simulink model "torch_3dof_angle"  (R2024a)
settings: Solver=FixedStepAuto  StartTime=0.0  StopTime=50  FixedStep=framePeriod_s  RelTol=1e-3
undefined symbols (not defined in the file): Aircraft, DiscIntNeverNeededParam, framePeriod_s, frameRate_hz, magnitude
libraries: simulink x36, slpidlib x11, dspmathops x1, simulink_extras x1
(part 3 of 4)

== system torch_3dof_angle/WAYPOINT CONTROLLER/WP_NAV/Subsystem ==
  Sys_input : Inport
  tar_pos : Inport  Port=2
  max_v_z_mps : Inport  Port=3
  Bus Selector : BusSelector  OutputSignals=StateEstData.aux_ins.ned_pos_m
  Cast To Single : DataTypeConversion  OutDataTypeStr=single  SaturateOnIntegerOverflow=off  RndMeth=Floor
  Selector : Selector  InputPortWidth=3  IndexOptions=Index vector (dialog)  Indices=3  OutputSizes=1
  Selector1 : Selector  InputPortWidth=3  IndexOptions=Index vector (dialog)  Indices=3  OutputSizes=1
  Vertical position controller1 : Subsystem
  ve_z_cmd_mps : Outport
  wires:
  Vertical position controller1/1(ve_z_cmd_mps) -> ve_z_cmd_mps/1  "ve_z_cmd_mps"
  tar_pos/1 -> Selector/1
  Sys_input/1 -> Bus Selector/1
  Bus Selector/1 -> Selector1/1  "<ned_pos_m>"
  Selector1/1 -> Cast To Single/1
  max_v_z_mps/1 -> Vertical position controller1/3(max_v_z_mps)
  Selector/1 -> Vertical position controller1/2(tar_z)
  Cast To Single/1 -> Vertical position controller1/1(cur_alt)

== system torch_3dof_angle/WAYPOINT CONTROLLER/WP_NAV/Vertical position controller ==
  Sys_input : Inport
  max_v_z_mps : Inport  Port=2
  cur_target_pos_m : Inport  Port=3
  Bus Selector6 : BusSelector  OutputSignals=Navigation Filter Data.bfs_ekf.ned_pos_m
  Selector1 : Selector  InputPortWidth=3  IndexOptions=Index vector (dialog)  Indices=3  OutputSizes=1
  select_cur_z : Selector  InputPortWidth=3  IndexOptions=Index vector (dialog)  Indices=3  OutputSizes=1
  vertical_position_controller : Subsystem
  ve_z_cmd_mps : Outport
  wires:
  Sys_input/1 -> Bus Selector6/1
  Bus Selector6/1 -> select_cur_z/1  "<ned_pos_m>"
  vertical_position_controller/1(ve_z_cmd) -> ve_z_cmd_mps/1
  Selector1/1 -> vertical_position_controller/1(target_z_m)  "target_z"
  select_cur_z/1 -> vertical_position_controller/2(cur_z_m)
  cur_target_pos_m/1 -> Selector1/1
  max_v_z_mps/1 -> vertical_position_controller/3(max_v_z_mps)

== system torch_3dof_angle/WAYPOINT CONTROLLER/WP_NAV/heading_controller ==
  Sys_input : Inport
  cur_target_heading_rad : Inport  Port=2
  Bus Selector4 : BusSelector  OutputSignals=Navigation Filter Data.bfs_ekf.heading_rad
  heading_controller : Subsystem
  yaw_rate_cmd_radps : Outport
  wires:
  Sys_input/1 -> Bus Selector4/1
  cur_target_heading_rad/1 -> heading_controller/1(heading_cmd_rad)
  Bus Selector4/1 -> heading_controller/2(<heading_rad>)  "<heading_rad>"
  heading_controller/1(yaw_rate_cmd) -> yaw_rate_cmd_radps/1

== system torch_3dof_angle/determine arm and mode selection/Failsafe_management/Radio failsafe ==
  note: Transition to RTL mode
  note: If radio_failsafe is triggered and current_mode is not auto, rtl, land nor motor_state disarmed then RTL mode is triggered
  failsafe : Inport
  manual_mode : Inport  Port=2
  motor_state : Inport  Port=3
  AND1 : Logic  Commented=on  IconShape=distinctive  AllPortsSameDT=off  OutDataTypeStr=boolean
  Compare To Constant : simulink/Logic and Bit Operations/Compare To Constant  Commented=on  relop=~=  const=3  OutDataTypeStr=boolean
  Compare To Constant1 : simulink/Logic and Bit Operations/Compare To Constant  Commented=on  relop=~=  const=4  OutDataTypeStr=boolean
  Compare To Constant2 : simulink/Logic and Bit Operations/Compare To Constant  Commented=on  relop=~=  const=5  OutDataTypeStr=boolean
  NOR : Logic  Commented=on  Operator=NOR  Inputs=4  IconShape=distinctive  AllPortsSameDT=off  OutDataTypeStr=boolean
  NOT : Logic  Commented=on  Operator=NOT  IconShape=distinctive  AllPortsSameDT=off  OutDataTypeStr=boolean
  NOT1 : Logic  Operator=NOT  IconShape=distinctive  AllPortsSameDT=off  OutDataTypeStr=boolean
  Subsystem : Subsystem
  radio_failsafe_enabled : Outport
  wires:
  manual_mode/1 -> Compare To Constant2/1, Compare To Constant1/1, Compare To Constant/1
  Compare To Constant/1 -> NOR/1
  Compare To Constant1/1 -> NOR/2
  Compare To Constant2/1 -> NOR/3
  motor_state/1 -> NOT/1
  NOT/1 -> NOR/4
  failsafe/1 -> Subsystem/1(<inceptor_health>)
  NOR/1 -> AND1/1
  Subsystem/1(inceptor_health_filtered) -> NOT1/1
  NOT1/1 -> radio_failsafe_enabled/1

== system torch_3dof_angle/determine arm and mode selection/Subsystem/e_stop counter ==
  note: This is to ensure e_stop event is not triggered unless e_stop command is sent for more than 0.3 s to prevent false trigger
  motor_e_stop_raw : Inport
  Enable : EnablePort  StatesWhenEnabling=reset
  Compare To Constant : simulink/Logic and Bit Operations/Compare To Constant  relop=>=  const=0.5  OutDataTypeStr=boolean
  Discrete-Time Integrator : DiscreteIntegrator  SampleTime=framePeriod_s  LimitOutput=on  UpperSaturationLimit=1  LowerSaturationLimit=0  ICPrevOutput=DiscIntNeverNeededParam  ICPrevScaledInput=DiscIntNeverNeededParam
  Gain : Gain  Gain=2
  e_stop_filtered : Outport
  wires:
  Compare To Constant/1 -> e_stop_filtered/1
  Discrete-Time Integrator/1 -> Compare To Constant/1
  Gain/1 -> Discrete-Time Integrator/1
  motor_e_stop_raw/1 -> Gain/1

== system torch_3dof_angle/determine arm and mode selection/yaw_stick_arming/Enabled Subsystem ==
  yaw_input : Inport
  Enable : EnablePort  StatesWhenEnabling=reset
  Cast : DataTypeConversion  OutDataTypeStr=int8  SaturateOnIntegerOverflow=off  RndMeth=Floor
  Discrete-Time Integrator : DiscreteIntegrator  IntegratorMethod=Integration: Trapezoidal  SampleTime=framePeriod_s  OutDataTypeStr=single  UpperSaturationLimit=1  LowerSaturationLimit=0  ICPrevOutput=DiscIntNeverNeededParam  ICPrevScaledInput=DiscIntNeverNeededParam
  time_arm_valid_s : Outport
  wires:
  Discrete-Time Integrator/1 -> time_arm_valid_s/1
  Cast/1 -> Discrete-Time Integrator/1
  yaw_input/1 -> Cast/1

== system torch_3dof_angle/determine arm and mode selection/yaw_stick_arming/manual_arming ==
  yaw_arm : Inport
  Trigger : TriggerPort  VariantControl=(inherit)  PortDimensions=1
  arm_state : Outport
  wires:
  yaw_arm/1 -> arm_state/1

== system torch_3dof_angle/POS_HOLD CONTROLLER/Horizontal speed controller/Subsystem/roll_D_DLPF ==
  raw_val : Inport
  freq_cut : Inport  Port=2
  Constant : Constant  Value=50  OutDataTypeStr=single
  MATLAB Function : MATLAB Function  TreatAsAtomicUnit=on
  Unit Delay : UnitDelay  SampleTime=-1  HasFrameUpgradeWarning=on
  filtered_val : Outport
  wires:
  freq_cut/1 -> MATLAB Function/3(freq_cut)
  MATLAB Function/1(filtered_val) -> Unit Delay/1, filtered_val/1
  Unit Delay/1 -> MATLAB Function/1(prev_val)
  raw_val/1 -> MATLAB Function/2(raw_val)
  Constant/1 -> MATLAB Function/4(samp_freq)

== system torch_3dof_angle/POS_HOLD CONTROLLER/Horizontal speed controller/Subsystem1/roll_D_DLPF ==
  raw_val : Inport
  freq_cut : Inport  Port=2
  Constant : Constant  Value=50  OutDataTypeStr=single
  MATLAB Function : MATLAB Function  TreatAsAtomicUnit=on
  Unit Delay : UnitDelay  SampleTime=-1  HasFrameUpgradeWarning=on
  filtered_val : Outport
  wires:
  freq_cut/1 -> MATLAB Function/3(freq_cut)
  MATLAB Function/1(filtered_val) -> Unit Delay/1, filtered_val/1
  Unit Delay/1 -> MATLAB Function/1(prev_val)
  raw_val/1 -> MATLAB Function/2(raw_val)
  Constant/1 -> MATLAB Function/4(samp_freq)

== system torch_3dof_angle/POS_HOLD CONTROLLER/Horizontal speed controller/zero_vel_handling/Horizontal position controller ==
  cur_target_pos_m : Inport
  cur_pos_m : Inport  Port=2
  P_xy : Inport  Port=3
  Horizontal_position_controller : Subsystem
  "horizontal_error_calculation " : Subsystem
  ve_xy : Outport
  dist_to_tar : Outport  Port=2
  bearing_to_tar : Outport  Port=3
  wires:
  Horizontal_position_controller/1(Ve_xy) -> ve_xy/1
  "horizontal_error_calculation "/1(dist_to_target_m) -> dist_to_tar/1, Horizontal_position_controller/1(dist_to_tar_m)
  "horizontal_error_calculation "/2(bearing_to_tar_rad) -> bearing_to_tar/1, Horizontal_position_controller/2(bearing_to_tar_rad)
  cur_target_pos_m/1 -> "horizontal_error_calculation "/1(target_pos_m)
  cur_pos_m/1 -> "horizontal_error_calculation "/2(cur_pos_m)
  P_xy/1 -> Horizontal_position_controller/3(gain)

== system torch_3dof_angle/POS_HOLD CONTROLLER/Horizontal speed controller/zero_vel_handling/delay_on_instant_off ==
  in : Inport
  AND : Logic  IconShape=distinctive  AllPortsSameDT=off  OutDataTypeStr=boolean
  delayed : Subsystem
  out : Outport
  wires:
  delayed/1(delayed_sig) -> AND/1
  in/1 -> AND/2, delayed/1(sig)
  AND/1 -> out/1

== system torch_3dof_angle/POS_HOLD CONTROLLER/Horizontal speed controller/zero_vel_handling/set_tar_pos when vel_cmd == 0 ==
  pos_xy_m : Inport
  Enable : EnablePort
  target_pos_xy_m : Outport
  wires:
  pos_xy_m/1 -> target_pos_xy_m/1

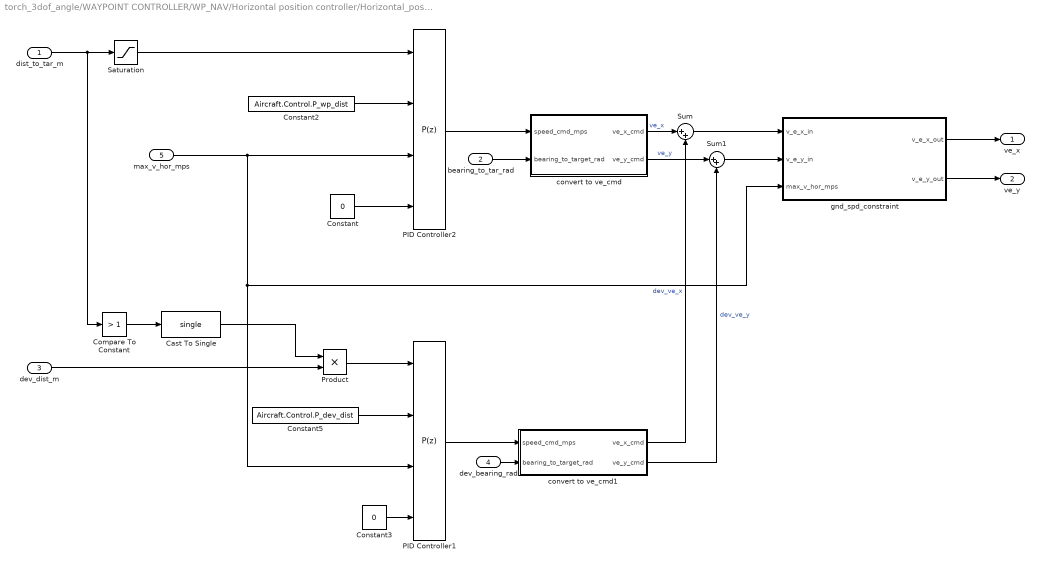
== system torch_3dof_angle/WAYPOINT CONTROLLER/WP_NAV/Horizontal position controller/Horizontal_position_controller ==
  dist_to_tar_m : Inport
  bearing_to_tar_rad : Inport  Port=2
  dev_dist_m : Inport  Port=3
  dev_bearing_rad : Inport  Port=4
  max_v_hor_mps : Inport  Port=5
  Cast To Single : DataTypeConversion  OutDataTypeStr=single  SaturateOnIntegerOverflow=off  RndMeth=Floor
  Compare To Constant : simulink/Logic and Bit Operations/Compare To Constant  relop=>  const=1  OutDataTypeStr=boolean
  Constant : Constant  Value=0  OutDataTypeStr=single
  Constant2 : Constant  Value=Aircraft.Control.P_wp_dist  OutDataTypeStr=single
  Constant3 : Constant  Value=0  OutDataTypeStr=single
  Constant5 : Constant  Value=Aircraft.Control.P_dev_dist  OutDataTypeStr=single
  PID Controller1 : slpidlib/PID Controller  Controller=P  Form=Parallel  TimeDomain=Discrete-time  UseExternalTs=off  SampleTime=framePeriod_s  IntegratorMethod=Forward Euler  FilterMethod=Forward Euler  ControllerParametersSource=external  P=0.335  I=0.005  UseKiTs=off  D=0  UseExternalDerivativeSource=off  N=100  UseFilter=off  TunerSelectOption=Transfer Function Based (PID Tuner App)  InitialConditionSource=internal  InitialConditionForIntegrator=0  InitialConditionForFilter=0  DifferentiatorICPrevScaledInput=0  ExternalReset=none  TrackingMode=off  Kt=1  LimitOutput=on  SatLimitsSource=external  UpperSaturationLimit=inf  LowerSaturationLimit=-inf  LinearizeAsGain=off  AntiWindupMode=clamping  Kb=1  LimitIntegrator=off  UpperIntegratorSaturationLimit=inf  LowerIntegratorSaturationLimit=-inf  POutMin=[]  POutMax=[]  IOutMin=[]  IOutMax=[]  DOutMin=[]  DOutMax=[]  NOutMin=[]  NOutMax=[]  SumOutMin=[]  SumOutMax=[]  SaturationOutMin=[]  SaturationOutMax=[]  PParamMin=[]  PParamMax=[]  IParamMin=[]  IParamMax=[]  DParamMin=[]  DParamMax=[]  NParamMin=[]  NParamMax=[]  KbParamMin=[]  KbParamMax=[]  KtParamMin=[]  KtParamMax=[]  KbOutMin=[]  KbOutMax=[]  KtOutMin=[]  KtOutMax=[]  IntegratorOutMin=[]  IntegratorOutMax=[]  FilterOutMin=[]  FilterOutMax=[]  SumI1OutMin=[]  SumI1OutMax=[]  SumI2OutMin=[]  SumI2OutMax=[]  SumI3OutMin=[]  SumI3OutMax=[]  SumI4OutMin=[]  SumI4OutMax=[]  SumDOutMin=[]  SumDOutMax=[]  DifferentiatorOutMin=[]  DifferentiatorOutMax=[]  FilterDiffOutCoefMin=[]  FilterDiffOutCoefMax=[]  ReciprocalOutMin=[]  ReciprocalOutMax=[]  SumDenOutMin=[]  SumDenOutMax=[]  SumNumOutMin=[]  SumNumOutMax=[]  DivideOutMin=[]  DivideOutMax=[]  UdiffTsProdOutMin=[]  UdiffTsProdOutMax=[]  NTsProdOutMin=[]  NTsProdOutMax=[]  UintegralTsProdOutMin=[]  UintegralTsProdOutMax=[]  UngainTsProdOutMin=[]  UngainTsProdOutMax=[]  ClampingZeroOutDataTypeStr=Inherit: Inherit via back propagation  ClampingZeroOutMin=[]  ClampingZeroOutMax=[]  FilterDenConstantOutDataTypeStr=Inherit: Inherit via back propagation  FilterDenConstantOutMin=[]  FilterDenConstantOutMax=[]  PCopyOutDataTypeStr=Inherit: Inherit via back propagation  PCopyOutMin=[]  PCopyOutMax=[]  NCopyOutDataTypeStr=Inherit: Inherit via back propagation  NCopyOutMin=[]  NCopyOutMax=[]  IntegratorContinuousStateAttributes=''  IntegratorStateMustResolveToSignalObject=off  IntegratorRTWStateStorageClass=Auto  FilterContinuousStateAttributes=''  FilterStateMustResolveToSignalObject=off  FilterRTWStateStorageClass=Auto  ParallelPVariant=ExternalParameters  IdealPVariant=Disabled  IVariant=Disabled  DVariant=Disabled  IntegratorVariant=Disabled  SatVariant=External  AWVariant=Disabled  PCopyVariant=Disabled  TRVariant=Disabled  FdbkBlocksVariant=Forward  IdealPFdbkVariant=Disabled  SatFdbkVariant=Disabled  DerivativeFilterVariant=Disabled  NVariant=Disabled  NCopyVariant=Disabled_SignalSpec  FilterICVariant=Disabled  IntegratorICVariant=Disabled  ExternalResetVariant=Disabled  TRSumVariant=Passthrough  SumFdbkVariant=Disabled  SumVariant=Passthrough_P  TsampFilterVariant=InternalTs  TsampNgainVariant=Passthrough  TsampIntegralVariant=Disabled_SignalSpec  ExternalSaturationOutDataTypeStr=Inherit: Same as second input  DerivativeSourceVariant=Disabled
  PID Controller2 : slpidlib/PID Controller  Controller=P  Form=Parallel  TimeDomain=Discrete-time  UseExternalTs=off  SampleTime=framePeriod_s  IntegratorMethod=Forward Euler  FilterMethod=Forward Euler  ControllerParametersSource=external  P=0.335  I=0.005  UseKiTs=off  D=0  UseExternalDerivativeSource=off  N=100  UseFilter=off  TunerSelectOption=Transfer Function Based (PID Tuner App)  InitialConditionSource=internal  InitialConditionForIntegrator=0  InitialConditionForFilter=0  DifferentiatorICPrevScaledInput=0  ExternalReset=none  TrackingMode=off  Kt=1  LimitOutput=on  SatLimitsSource=external  UpperSaturationLimit=inf  LowerSaturationLimit=-inf  LinearizeAsGain=off  AntiWindupMode=clamping  Kb=1  LimitIntegrator=off  UpperIntegratorSaturationLimit=inf  LowerIntegratorSaturationLimit=-inf  POutMin=[]  POutMax=[]  IOutMin=[]  IOutMax=[]  DOutMin=[]  DOutMax=[]  NOutMin=[]  NOutMax=[]  SumOutMin=[]  SumOutMax=[]  SaturationOutMin=[]  SaturationOutMax=[]  PParamMin=[]  PParamMax=[]  IParamMin=[]  IParamMax=[]  DParamMin=[]  DParamMax=[]  NParamMin=[]  NParamMax=[]  KbParamMin=[]  KbParamMax=[]  KtParamMin=[]  KtParamMax=[]  KbOutMin=[]  KbOutMax=[]  KtOutMin=[]  KtOutMax=[]  IntegratorOutMin=[]  IntegratorOutMax=[]  FilterOutMin=[]  FilterOutMax=[]  SumI1OutMin=[]  SumI1OutMax=[]  SumI2OutMin=[]  SumI2OutMax=[]  SumI3OutMin=[]  SumI3OutMax=[]  SumI4OutMin=[]  SumI4OutMax=[]  SumDOutMin=[]  SumDOutMax=[]  DifferentiatorOutMin=[]  DifferentiatorOutMax=[]  FilterDiffOutCoefMin=[]  FilterDiffOutCoefMax=[]  ReciprocalOutMin=[]  ReciprocalOutMax=[]  SumDenOutMin=[]  SumDenOutMax=[]  SumNumOutMin=[]  SumNumOutMax=[]  DivideOutMin=[]  DivideOutMax=[]  UdiffTsProdOutMin=[]  UdiffTsProdOutMax=[]  NTsProdOutMin=[]  NTsProdOutMax=[]  UintegralTsProdOutMin=[]  UintegralTsProdOutMax=[]  UngainTsProdOutMin=[]  UngainTsProdOutMax=[]  ClampingZeroOutDataTypeStr=Inherit: Inherit via back propagation  ClampingZeroOutMin=[]  ClampingZeroOutMax=[]  FilterDenConstantOutDataTypeStr=Inherit: Inherit via back propagation  FilterDenConstantOutMin=[]  FilterDenConstantOutMax=[]  PCopyOutDataTypeStr=Inherit: Inherit via back propagation  PCopyOutMin=[]  PCopyOutMax=[]  NCopyOutDataTypeStr=Inherit: Inherit via back propagation  NCopyOutMin=[]  NCopyOutMax=[]  IntegratorContinuousStateAttributes=''  IntegratorStateMustResolveToSignalObject=off  IntegratorRTWStateStorageClass=Auto  FilterContinuousStateAttributes=''  FilterStateMustResolveToSignalObject=off  FilterRTWStateStorageClass=Auto  ParallelPVariant=ExternalParameters  IdealPVariant=Disabled  IVariant=Disabled  DVariant=Disabled  IntegratorVariant=Disabled  SatVariant=External  AWVariant=Disabled  PCopyVariant=Disabled  TRVariant=Disabled  FdbkBlocksVariant=Forward  IdealPFdbkVariant=Disabled  SatFdbkVariant=Disabled  DerivativeFilterVariant=Disabled  NVariant=Disabled  NCopyVariant=Disabled_SignalSpec  FilterICVariant=Disabled  IntegratorICVariant=Disabled  ExternalResetVariant=Disabled  TRSumVariant=Passthrough  SumFdbkVariant=Disabled  SumVariant=Passthrough_P  TsampFilterVariant=InternalTs  TsampNgainVariant=Passthrough  TsampIntegralVariant=Disabled_SignalSpec  ExternalSaturationOutDataTypeStr=Inherit: Same as second input  DerivativeSourceVariant=Disabled
  Product : Product
  Saturation : Saturate  UpperLimit=1  LowerLimit=0
  Sum : Sum  Inputs=|++
  Sum1 : Sum  Inputs=|++
  convert to ve_cmd : Subsystem
  convert to ve_cmd1 : Subsystem
  "gnd_spd_constraint " : Subsystem
  ve_x : Outport
  ve_y : Outport  Port=2
  wires:
  Constant2/1 -> PID Controller2/2
  bearing_to_tar_rad/1 -> convert to ve_cmd/2(bearing_to_target_rad)
  Constant/1 -> PID Controller2/4
  Saturation/1 -> PID Controller2/1
  PID Controller2/1 -> convert to ve_cmd/1(speed_cmd_mps)
  "gnd_spd_constraint "/1(v_e_x_out) -> ve_x/1
  "gnd_spd_constraint "/2(v_e_y_out) -> ve_y/1
  PID Controller1/1 -> convert to ve_cmd1/1(speed_cmd_mps)
  dev_bearing_rad/1 -> convert to ve_cmd1/2(bearing_to_target_rad)
  Constant3/1 -> PID Controller1/4
  max_v_hor_mps/1 -> PID Controller1/3, "gnd_spd_constraint "/3(max_v_hor_mps), PID Controller2/3
  convert to ve_cmd/1(ve_x_cmd) -> Sum/1  "ve_x"
  convert to ve_cmd/2(ve_y_cmd) -> Sum1/1  "ve_y"
  convert to ve_cmd1/1(ve_x_cmd) -> Sum/2  "dev_ve_x"
  convert to ve_cmd1/2(ve_y_cmd) -> Sum1/2  "dev_ve_y"
  Sum1/1 -> "gnd_spd_constraint "/2(v_e_y_in)
  Sum/1 -> "gnd_spd_constraint "/1(v_e_x_in)
  Constant5/1 -> PID Controller1/2
  dist_to_tar_m/1 -> Saturation/1, Compare To Constant/1
  Compare To Constant/1 -> Cast To Single/1
  Cast To Single/1 -> Product/1
  dev_dist_m/1 -> Product/2
  Product/1 -> PID Controller1/1

== system torch_3dof_angle/WAYPOINT CONTROLLER/WP_NAV/Horizontal position controller/horizontal_error_calculation  ==
  target_pos_m : Inport
  cur_pos_m : Inport  Port=2
  Atan2 : Trigonometry  Operator=atan2
  Cast To Single : DataTypeConversion  OutDataTypeStr=single  SaturateOnIntegerOverflow=off  RndMeth=Floor
  Cast To Single1 : DataTypeConversion  OutDataTypeStr=single  SaturateOnIntegerOverflow=off  RndMeth=Floor
  Demux2 : Demux  Outputs=2
  MatrixMultiply : Product  Multiplication=Matrix(*)
  Selector : Selector  InputPortWidth=3  IndexOptions=Index vector (dialog)  Indices=[1 2]  OutputSizes=1
  Sqrt : Sqrt
  Subtract : Sum  Inputs=+-
  Transpose : Math  Operator=transpose
  dist_to_target_m : Outport
  bearing_to_tar_rad : Outport  Port=2
  wires:
  target_pos_m/1 -> Subtract/1
  cur_pos_m/1 -> Subtract/2
  Selector/1 -> Demux2/1, MatrixMultiply/2, Transpose/1
  Atan2/1 -> Cast To Single1/1
  Subtract/1 -> Selector/1
  Demux2/2 -> Atan2/1
  Transpose/1 -> MatrixMultiply/1
  MatrixMultiply/1 -> Sqrt/1
  Demux2/1 -> Atan2/2
  Sqrt/1 -> Cast To Single/1
  Cast To Single/1 -> dist_to_target_m/1
  Cast To Single1/1 -> bearing_to_tar_rad/1

== system torch_3dof_angle/WAYPOINT CONTROLLER/WP_NAV/Subsystem/Vertical position controller1 ==
  cur_alt : Inport
  tar_z : Inport  Port=2
  max_v_z_mps : Inport  Port=3
  Altitude PID : slpidlib/PID Controller  Controller=P  Form=Ideal  TimeDomain=Discrete-time  UseExternalTs=off  SampleTime=framePeriod_s  IntegratorMethod=Forward Euler  FilterMethod=Forward Euler  ControllerParametersSource=external  P=0  I=0  UseKiTs=off  D=0  UseExternalDerivativeSource=off  N=100  UseFilter=off  TunerSelectOption=Frequency Response Based  ZeroCross=off  InitialConditionSource=internal  InitialConditionForIntegrator=0  InitialConditionForFilter=0  DifferentiatorICPrevScaledInput=0  ExternalReset=either  TrackingMode=off  Kt=1  LimitOutput=on  SatLimitsSource=external  UpperSaturationLimit=Aircraft.Control.v_z_max  LowerSaturationLimit=-Aircraft.Control.v_z_max  LinearizeAsGain=on  AntiWindupMode=clamping  Kb=1  LimitIntegrator=off  UpperIntegratorSaturationLimit=inf  LowerIntegratorSaturationLimit=-inf  POutMin=[]  POutMax=[]  IOutMin=[]  IOutMax=[]  DOutMin=[]  DOutMax=[]  NOutMin=[]  NOutMax=[]  SumOutMin=[]  SumOutMax=[]  SaturationOutMin=[]  SaturationOutMax=[]  PParamMin=[]  PParamMax=[]  IParamMin=[]  IParamMax=[]  DParamMin=[]  DParamMax=[]  NParamMin=[]  NParamMax=[]  KbParamMin=[]  KbParamMax=[]  KtParamMin=[]  KtParamMax=[]  KbOutMin=[]  KbOutMax=[]  KtOutMin=[]  KtOutMax=[]  IntegratorOutMin=[]  IntegratorOutMax=[]  FilterOutMin=[]  FilterOutMax=[]  SumI1OutMin=[]  SumI1OutMax=[]  SumI2OutMin=[]  SumI2OutMax=[]  SumI3OutMin=[]  SumI3OutMax=[]  SumI4OutMin=[]  SumI4OutMax=[]  SumDOutMin=[]  SumDOutMax=[]  DifferentiatorOutMin=[]  DifferentiatorOutMax=[]  FilterDiffOutCoefMin=[]  FilterDiffOutCoefMax=[]  ReciprocalOutMin=[]  ReciprocalOutMax=[]  SumDenOutMin=[]  SumDenOutMax=[]  SumNumOutMin=[]  SumNumOutMax=[]  DivideOutMin=[]  DivideOutMax=[]  UdiffTsProdOutMin=[]  UdiffTsProdOutMax=[]  NTsProdOutMin=[]  NTsProdOutMax=[]  UintegralTsProdOutMin=[]  UintegralTsProdOutMax=[]  UngainTsProdOutMin=[]  UngainTsProdOutMax=[]  ClampingZeroOutDataTypeStr=Inherit: Inherit via back propagation  ClampingZeroOutMin=[]  ClampingZeroOutMax=[]  FilterDenConstantOutDataTypeStr=Inherit: Inherit via back propagation  FilterDenConstantOutMin=[]  FilterDenConstantOutMax=[]  PCopyOutDataTypeStr=Inherit: Inherit via back propagation  PCopyOutMin=[]  PCopyOutMax=[]  NCopyOutDataTypeStr=Inherit: Inherit via back propagation  NCopyOutMin=[]  NCopyOutMax=[]  IntegratorContinuousStateAttributes=''  IntegratorStateMustResolveToSignalObject=off  IntegratorRTWStateStorageClass=Auto  FilterContinuousStateAttributes=''  FilterStateMustResolveToSignalObject=off  FilterRTWStateStorageClass=Auto  ParallelPVariant=ExternalParameters  IdealPVariant=Disabled  IVariant=Disabled  DVariant=Disabled  IntegratorVariant=Disabled  SatVariant=External  AWVariant=Disabled  PCopyVariant=Disabled  TRVariant=Disabled  FdbkBlocksVariant=Forward  IdealPFdbkVariant=Disabled  SatFdbkVariant=Disabled  DerivativeFilterVariant=Disabled  NVariant=Disabled  NCopyVariant=Disabled_SignalSpec  FilterICVariant=Disabled  IntegratorICVariant=Disabled  ExternalResetVariant=Disabled  TRSumVariant=Passthrough  SumFdbkVariant=Disabled  SumVariant=Passthrough_P  TsampFilterVariant=InternalTs  TsampNgainVariant=Passthrough  TsampIntegralVariant=Disabled_SignalSpec  ExternalSaturationOutDataTypeStr=Inherit: Same as second input  DerivativeSourceVariant=Disabled
  Constant3 : Constant  Value=Aircraft.Control.P_alt  OutDataTypeStr=single
  Gain : Gain  Gain=-1
  Sum3 : Sum  Inputs=|+-
  ve_z_cmd_mps : Outport
  wires:
  Altitude PID/1 -> ve_z_cmd_mps/1
  tar_z/1 -> Sum3/1  "target_z"
  cur_alt/1 -> Sum3/2
  Sum3/1 -> Altitude PID/1
  Constant3/1 -> Altitude PID/2
  max_v_z_mps/1 -> Gain/1, Altitude PID/3
  Gain/1 -> Altitude PID/4

== system torch_3dof_angle/WAYPOINT CONTROLLER/WP_NAV/Vertical position controller/vertical_position_controller ==
  target_z_m : Inport
  cur_z_m : Inport  Port=2
  max_v_z_mps : Inport  Port=3
  Altitude PID : slpidlib/PID Controller  Controller=PI  Form=Ideal  TimeDomain=Discrete-time  UseExternalTs=off  SampleTime=framePeriod_s  IntegratorMethod=Forward Euler  FilterMethod=Forward Euler  ControllerParametersSource=external  P=0  I=0  UseKiTs=off  D=0  N=100  UseFilter=off  TunerSelectOption=Frequency Response Based  ZeroCross=off  InitialConditionSource=internal  InitialConditionForIntegrator=0  InitialConditionForFilter=0  DifferentiatorICPrevScaledInput=0  ExternalReset=none  TrackingMode=off  Kt=1  LimitOutput=on  SatLimitsSource=external  UpperSaturationLimit=Aircraft.Control.v_z_up_max  LowerSaturationLimit=-Aircraft.Control.v_z_down_max  LinearizeAsGain=on  AntiWindupMode=clamping  Kb=1  POutMin=[]  POutMax=[]  IOutMin=[]  IOutMax=[]  DOutMin=[]  DOutMax=[]  NOutMin=[]  NOutMax=[]  SumOutMin=[]  SumOutMax=[]  SaturationOutMin=[]  SaturationOutMax=[]  PParamMin=[]  PParamMax=[]  IParamMin=[]  IParamMax=[]  DParamMin=[]  DParamMax=[]  NParamMin=[]  NParamMax=[]  KbParamMin=[]  KbParamMax=[]  KtParamMin=[]  KtParamMax=[]  KbOutMin=[]  KbOutMax=[]  KtOutMin=[]  KtOutMax=[]  IntegratorOutMin=[]  IntegratorOutMax=[]  FilterOutMin=[]  FilterOutMax=[]  SumI1OutMin=[]  SumI1OutMax=[]  SumI2OutMin=[]  SumI2OutMax=[]  SumI3OutMin=[]  SumI3OutMax=[]  SumI4OutMin=[]  SumI4OutMax=[]  SumDOutMin=[]  SumDOutMax=[]  DifferentiatorOutMin=[]  DifferentiatorOutMax=[]  FilterDiffOutCoefMin=[]  FilterDiffOutCoefMax=[]  ReciprocalOutMin=[]  ReciprocalOutMax=[]  SumDenOutMin=[]  SumDenOutMax=[]  SumNumOutMin=[]  SumNumOutMax=[]  DivideOutMin=[]  DivideOutMax=[]  UdiffTsProdOutMin=[]  UdiffTsProdOutMax=[]  NTsProdOutMin=[]  NTsProdOutMax=[]  UintegralTsProdOutMin=[]  UintegralTsProdOutMax=[]  UngainTsProdOutMin=[]  UngainTsProdOutMax=[]  IntegratorContinuousStateAttributes=''  IntegratorStateMustResolveToSignalObject=off  IntegratorRTWStateStorageClass=Auto  FilterContinuousStateAttributes=''  FilterStateMustResolveToSignalObject=off  FilterRTWStateStorageClass=Auto  ParallelPVariant=Passthrough  IdealPVariant=ExternalParameters  IVariant=ExternalParameters  DVariant=Disabled  IntegratorVariant=Discrete  SatVariant=External  AWVariant=DiscClampingIdeal  PCopyVariant=ExternalParamsIdeal  TRVariant=Disabled  FdbkBlocksVariant=Forward  IdealPFdbkVariant=Disabled  SatFdbkVariant=Disabled  DerivativeFilterVariant=Disabled  NVariant=Disabled  NCopyVariant=Disabled_SignalSpec  FilterICVariant=Disabled  IntegratorICVariant=InternalICs  ExternalResetVariant=Disabled  TRSumVariant=Passthrough  SumFdbkVariant=Disabled  SumVariant=Sum_PI  TsampFilterVariant=InternalTs  TsampNgainVariant=Passthrough  TsampIntegralVariant=Passthrough  ExternalSaturationOutDataTypeStr=Inherit: Same as second input  aMode=0
  Constant : Constant  Value=Aircraft.Control.v_z_up_max  OutDataTypeStr=single
  Constant1 : Constant  Value=Aircraft.Control.v_z_down_max  OutDataTypeStr=single
  Gain : Gain  Gain=-1
  Min : MinMax  Inputs=2
  P_alt : Constant  Value=Aircraft.Control.P_alt  OutDataTypeStr=single
  P_alt1 : Constant  Value=Aircraft.Control.I_alt  OutDataTypeStr=single
  Sum3 : Sum  Inputs=|+-
  ve_z_cmd : Outport
  wires:
  P_alt/1 -> Altitude PID/2
  Sum3/1 -> Altitude PID/1
  max_v_z_mps/1 -> Min/1
  Constant/1 -> Min/2
  Constant1/1 -> Altitude PID/4
  Min/1 -> Gain/1
  Gain/1 -> Altitude PID/5
  P_alt1/1 -> Altitude PID/3
  Altitude PID/1 -> ve_z_cmd/1
  target_z_m/1 -> Sum3/1
  cur_z_m/1 -> Sum3/2

== system torch_3dof_angle/WAYPOINT CONTROLLER/WP_NAV/heading_controller/heading_controller ==
  heading_cmd_rad : Inport
  <heading_rad> : Inport  Port=2
  D_heading : Constant  Value=Aircraft.Control.D_heading  OutDataTypeStr=single
  Discrete Derivative : simulink/Discrete/Discrete Derivative  gainval=1.0  ICPrevScaledInput=0.0  OutMin=[]  OutMax=[]  OutDataType=fixdt(1, 16)  OutScaling=2^-10  DoSatur=off
  I_heading : Constant  Value=Aircraft.Control.I_heading  OutDataTypeStr=single
  PID Controller2 : slpidlib/PID Controller  Controller=PI  Form=Ideal  TimeDomain=Discrete-time  UseExternalTs=off  SampleTime=framePeriod_s  IntegratorMethod=Forward Euler  FilterMethod=Forward Euler  ControllerParametersSource=external  P=1.85  I=0.01  UseKiTs=off  D=0  N=100  UseFilter=off  TunerSelectOption=Transfer Function Based (PID Tuner App)  InitialConditionSource=internal  InitialConditionForIntegrator=0  InitialConditionForFilter=0  DifferentiatorICPrevScaledInput=0  ExternalReset=none  TrackingMode=off  Kt=1  LimitOutput=on  SatLimitsSource=internal  UpperSaturationLimit=inf  LowerSaturationLimit=-inf  LinearizeAsGain=on  AntiWindupMode=clamping  Kb=2  POutMin=[]  POutMax=[]  IOutMin=[]  IOutMax=[]  DOutMin=[]  DOutMax=[]  NOutMin=[]  NOutMax=[]  SumOutMin=[]  SumOutMax=[]  SaturationOutMin=[]  SaturationOutMax=[]  PParamMin=[]  PParamMax=[]  IParamMin=[]  IParamMax=[]  DParamMin=[]  DParamMax=[]  NParamMin=[]  NParamMax=[]  KbParamMin=[]  KbParamMax=[]  KtParamMin=[]  KtParamMax=[]  KbOutMin=[]  KbOutMax=[]  KtOutMin=[]  KtOutMax=[]  IntegratorOutMin=[]  IntegratorOutMax=[]  FilterOutMin=[]  FilterOutMax=[]  SumI1OutMin=[]  SumI1OutMax=[]  SumI2OutMin=[]  SumI2OutMax=[]  SumI3OutMin=[]  SumI3OutMax=[]  SumI4OutMin=[]  SumI4OutMax=[]  SumDOutMin=[]  SumDOutMax=[]  DifferentiatorOutMin=[]  DifferentiatorOutMax=[]  FilterDiffOutCoefMin=[]  FilterDiffOutCoefMax=[]  ReciprocalOutMin=[]  ReciprocalOutMax=[]  SumDenOutMin=[]  SumDenOutMax=[]  SumNumOutMin=[]  SumNumOutMax=[]  DivideOutMin=[]  DivideOutMax=[]  UdiffTsProdOutMin=[]  UdiffTsProdOutMax=[]  NTsProdOutMin=[]  NTsProdOutMax=[]  UintegralTsProdOutMin=[]  UintegralTsProdOutMax=[]  UngainTsProdOutMin=[]  UngainTsProdOutMax=[]  IntegratorContinuousStateAttributes=''  IntegratorStateMustResolveToSignalObject=off  IntegratorRTWStateStorageClass=Auto  FilterContinuousStateAttributes=''  FilterStateMustResolveToSignalObject=off  FilterRTWStateStorageClass=Auto  ParallelPVariant=Passthrough  IdealPVariant=ExternalParameters  IVariant=ExternalParameters  DVariant=Disabled  IntegratorVariant=Discrete  SatVariant=Enabled  AWVariant=DiscClampingIdeal  PCopyVariant=ExternalParamsIdeal  TRVariant=Disabled  FdbkBlocksVariant=Forward  IdealPFdbkVariant=Disabled  SatFdbkVariant=Disabled  DerivativeFilterVariant=Disabled  NVariant=Disabled  NCopyVariant=Disabled_SignalSpec  FilterICVariant=Disabled  IntegratorICVariant=InternalICs  ExternalResetVariant=Disabled  TRSumVariant=Passthrough  SumFdbkVariant=Disabled  SumVariant=Sum_PI  TsampFilterVariant=InternalTs  TsampNgainVariant=Passthrough  TsampIntegralVariant=Passthrough  ExternalSaturationOutDataTypeStr=Inherit: Same as second input  aMode=0
  P_heading : Constant  Value=Aircraft.Control.P_heading  OutDataTypeStr=single
  Product : Product
  Saturation : Saturate  UpperLimit=Aircraft.Control.yaw_rate_max  LowerLimit=-Aircraft.Control.yaw_rate_max
  Sum : Sum  Inputs=|+-
  heading_error : Subsystem
  yaw_rate_cmd : Outport
  wires:
  P_heading/1 -> PID Controller2/2
  heading_cmd_rad/1 -> heading_error/1(heading_cmd_rad)
  I_heading/1 -> PID Controller2/3
  <heading_rad>/1 -> Discrete Derivative/1, heading_error/2(heading_rad)
  Saturation/1 -> yaw_rate_cmd/1
  heading_error/1(heading_error_rad) -> PID Controller2/1
  Discrete Derivative/1 -> Product/1
  D_heading/1 -> Product/2
  PID Controller2/1 -> Sum/1
  Sum/1 -> Saturation/1
  Product/1 -> Sum/2

== system torch_3dof_angle/determine arm and mode selection/Failsafe_management/Radio failsafe/Subsystem ==
  <inceptor_health> : Inport
  Add : Sum
  Cast To Single : DataTypeConversion  OutDataTypeStr=single  SaturateOnIntegerOverflow=off  RndMeth=Floor
  Constant : Constant  Value=-0.5
  Gain : Gain  Gain=2
  Subsystem : Subsystem
  inceptor_health_filtered : Outport
  wires:
  Subsystem/1(incept_health_filter) -> inceptor_health_filtered/1
  <inceptor_health>/1 -> Cast To Single/1
  Cast To Single/1 -> Add/1
  Constant/1 -> Add/2
  Gain/1 -> Subsystem/1(<incept_health_raw>)
  Add/1 -> Gain/1

== system torch_3dof_angle/POS_HOLD CONTROLLER/Horizontal speed controller/zero_vel_handling/Horizontal position controller/Horizontal_position_controller ==
  dist_to_tar_m : Inport
  bearing_to_tar_rad : Inport  Port=2
  gain : Inport  Port=3
  Constant : Constant  Value=0  OutDataTypeStr=single
  Constant1 : Constant  Value=Aircraft.Control.v_hor_max  OutDataTypeStr=single
  Mux : Mux  Inputs=2
  PID Controller2 : slpidlib/PID Controller  Controller=P  Form=Parallel  TimeDomain=Discrete-time  UseExternalTs=off  SampleTime=framePeriod_s  IntegratorMethod=Forward Euler  FilterMethod=Forward Euler  ControllerParametersSource=external  P=0.335  I=0.005  UseKiTs=off  D=0  UseExternalDerivativeSource=off  N=100  UseFilter=off  TunerSelectOption=Transfer Function Based (PID Tuner App)  InitialConditionSource=internal  InitialConditionForIntegrator=0  InitialConditionForFilter=0  DifferentiatorICPrevScaledInput=0  ExternalReset=none  TrackingMode=off  Kt=1  LimitOutput=on  SatLimitsSource=external  UpperSaturationLimit=inf  LowerSaturationLimit=-inf  LinearizeAsGain=off  AntiWindupMode=clamping  Kb=1  LimitIntegrator=off  UpperIntegratorSaturationLimit=inf  LowerIntegratorSaturationLimit=-inf  POutMin=[]  POutMax=[]  IOutMin=[]  IOutMax=[]  DOutMin=[]  DOutMax=[]  NOutMin=[]  NOutMax=[]  SumOutMin=[]  SumOutMax=[]  SaturationOutMin=[]  SaturationOutMax=[]  PParamMin=[]  PParamMax=[]  IParamMin=[]  IParamMax=[]  DParamMin=[]  DParamMax=[]  NParamMin=[]  NParamMax=[]  KbParamMin=[]  KbParamMax=[]  KtParamMin=[]  KtParamMax=[]  KbOutMin=[]  KbOutMax=[]  KtOutMin=[]  KtOutMax=[]  IntegratorOutMin=[]  IntegratorOutMax=[]  FilterOutMin=[]  FilterOutMax=[]  SumI1OutMin=[]  SumI1OutMax=[]  SumI2OutMin=[]  SumI2OutMax=[]  SumI3OutMin=[]  SumI3OutMax=[]  SumI4OutMin=[]  SumI4OutMax=[]  SumDOutMin=[]  SumDOutMax=[]  DifferentiatorOutMin=[]  DifferentiatorOutMax=[]  FilterDiffOutCoefMin=[]  FilterDiffOutCoefMax=[]  ReciprocalOutMin=[]  ReciprocalOutMax=[]  SumDenOutMin=[]  SumDenOutMax=[]  SumNumOutMin=[]  SumNumOutMax=[]  DivideOutMin=[]  DivideOutMax=[]  UdiffTsProdOutMin=[]  UdiffTsProdOutMax=[]  NTsProdOutMin=[]  NTsProdOutMax=[]  UintegralTsProdOutMin=[]  UintegralTsProdOutMax=[]  UngainTsProdOutMin=[]  UngainTsProdOutMax=[]  ClampingZeroOutDataTypeStr=Inherit: Inherit via back propagation  ClampingZeroOutMin=[]  ClampingZeroOutMax=[]  FilterDenConstantOutDataTypeStr=Inherit: Inherit via back propagation  FilterDenConstantOutMin=[]  FilterDenConstantOutMax=[]  PCopyOutDataTypeStr=Inherit: Inherit via back propagation  PCopyOutMin=[]  PCopyOutMax=[]  NCopyOutDataTypeStr=Inherit: Inherit via back propagation  NCopyOutMin=[]  NCopyOutMax=[]  IntegratorContinuousStateAttributes=''  IntegratorStateMustResolveToSignalObject=off  IntegratorRTWStateStorageClass=Auto  FilterContinuousStateAttributes=''  FilterStateMustResolveToSignalObject=off  FilterRTWStateStorageClass=Auto  ParallelPVariant=ExternalParameters  IdealPVariant=Disabled  IVariant=Disabled  DVariant=Disabled  IntegratorVariant=Disabled  SatVariant=External  AWVariant=Disabled  PCopyVariant=Disabled  TRVariant=Disabled  FdbkBlocksVariant=Forward  IdealPFdbkVariant=Disabled  SatFdbkVariant=Disabled  DerivativeFilterVariant=Disabled  NVariant=Disabled  NCopyVariant=Disabled_SignalSpec  FilterICVariant=Disabled  IntegratorICVariant=Disabled  ExternalResetVariant=Disabled  TRSumVariant=Passthrough  SumFdbkVariant=Disabled  SumVariant=Passthrough_P  TsampFilterVariant=InternalTs  TsampNgainVariant=Passthrough  TsampIntegralVariant=Disabled_SignalSpec  ExternalSaturationOutDataTypeStr=Inherit: Same as second input  DerivativeSourceVariant=Disabled
  Saturation : Saturate  UpperLimit=1  LowerLimit=0
  convert to ve_cmd : Subsystem
  Ve_xy : Outport
  wires:
  bearing_to_tar_rad/1 -> convert to ve_cmd/2(bearing_to_target_rad)
  convert to ve_cmd/1(ve_x_cmd) -> Mux/1  "ve_x"
  convert to ve_cmd/2(ve_y_cmd) -> Mux/2  "ve_y"
  Mux/1 -> Ve_xy/1
  Constant1/1 -> PID Controller2/3
  Constant/1 -> PID Controller2/4
  Saturation/1 -> PID Controller2/1
  dist_to_tar_m/1 -> Saturation/1
  gain/1 -> PID Controller2/2
  PID Controller2/1 -> convert to ve_cmd/1(speed_cmd_mps)

== system torch_3dof_angle/POS_HOLD CONTROLLER/Horizontal speed controller/zero_vel_handling/Horizontal position controller/horizontal_error_calculation  ==
  target_pos_m : Inport
  cur_pos_m : Inport  Port=2
  Atan2 : Trigonometry  Operator=atan2
  Cast To Single : DataTypeConversion  OutDataTypeStr=single  SaturateOnIntegerOverflow=off  RndMeth=Floor
  Cast To Single1 : DataTypeConversion  OutDataTypeStr=single  SaturateOnIntegerOverflow=off  RndMeth=Floor
  Demux2 : Demux  Outputs=2
  MatrixMultiply : Product  Multiplication=Matrix(*)
  Sqrt : Sqrt
  Subtract : Sum  Inputs=+-
  Transpose : Math  Operator=transpose
  dist_to_target_m : Outport
  bearing_to_tar_rad : Outport  Port=2
  wires:
  target_pos_m/1 -> Subtract/1
  cur_pos_m/1 -> Subtract/2
  Subtract/1 -> Demux2/1, MatrixMultiply/2, Transpose/1
  Atan2/1 -> Cast To Single/1
  Demux2/2 -> Atan2/1
  Transpose/1 -> MatrixMultiply/1
  MatrixMultiply/1 -> Sqrt/1
  Demux2/1 -> Atan2/2
  Sqrt/1 -> Cast To Single1/1
  Cast To Single/1 -> bearing_to_tar_rad/1
  Cast To Single1/1 -> dist_to_target_m/1

== system torch_3dof_angle/POS_HOLD CONTROLLER/Horizontal speed controller/zero_vel_handling/delay_on_instant_off/delayed ==
  sig : Inport
  Constant : Constant  Value=framePeriod_s  OutDataTypeStr=single
  Constant1 : Constant  OutDataTypeStr=single
  Delay : Delay  DelayLengthSource=Input port  DelayLengthUpperLimit=10000
      settings: InputPortMap=u0,p1
  Divide : Product  Inputs=*/
  delayed_sig : Outport
  wires:
  Delay/1 -> delayed_sig/1
  sig/1 -> Delay/1
  Divide/1 -> Delay/2
  Constant/1 -> Divide/2
  Constant1/1 -> Divide/1

== system torch_3dof_angle/WAYPOINT CONTROLLER/WP_NAV/Horizontal position controller/Horizontal_position_controller/convert to ve_cmd ==
  speed_cmd_mps : Inport
  bearing_to_target_rad : Inport  Port=2
  Cos : Trigonometry  Operator=cos
  Product : Product
  Product1 : Product
  Sin : Trigonometry
  ve_x_cmd : Outport
  ve_y_cmd : Outport  Port=2
  wires:
  Product/1 -> ve_x_cmd/1
  speed_cmd_mps/1 -> Product/1, Product1/1
  bearing_to_target_rad/1 -> Cos/1, Sin/1
  Cos/1 -> Product/2
  Sin/1 -> Product1/2
  Product1/1 -> ve_y_cmd/1

== system torch_3dof_angle/WAYPOINT CONTROLLER/WP_NAV/Horizontal position controller/Horizontal_position_controller/convert to ve_cmd1 ==
  speed_cmd_mps : Inport
  bearing_to_target_rad : Inport  Port=2
  Cos : Trigonometry  Operator=cos
  Product : Product
  Product1 : Product
  Sin : Trigonometry
  ve_x_cmd : Outport
  ve_y_cmd : Outport  Port=2
  wires:
  Product/1 -> ve_x_cmd/1
  speed_cmd_mps/1 -> Product/1, Product1/1
  bearing_to_target_rad/1 -> Cos/1, Sin/1
  Cos/1 -> Product/2
  Sin/1 -> Product1/2
  Product1/1 -> ve_y_cmd/1

== system torch_3dof_angle/WAYPOINT CONTROLLER/WP_NAV/Horizontal position controller/Horizontal_position_controller/gnd_spd_constraint  ==
  v_e_x_in : Inport
  v_e_y_in : Inport  Port=2
  max_v_hor_mps : Inport  Port=3
  Demux : Demux  Outputs=2
  Magnitude Squared : Math  Operator=magnitude^2
  Mux : Mux  Inputs=2
  Normalization1 : dspmathops/Normalization  NormType=2-norm  Bias=1e-10  NormOver=Each column  Dimension=1  roundingMode=Floor  overflowMode=off  accumDataTypeStr=Inherit: Same as product output  accumLastDataTypeStr=Inherit: Same as product output  outputDataTypeStr=Inherit: Same as product output  outputMin=[]  outputMax=[]  outputLastDataTypeStr=Inherit: Same as product output
  Product : Product
  Sqrt : Sqrt
  Subtract : Sum  Inputs=-+
  Sum of Elements : Sum  Inputs=+
  Switch : Switch  Criteria=u2 > Threshold  SaturateOnIntegerOverflow=off  InputSameDT=off
  v_e_x_out : Outport
  v_e_y_out : Outport  Port=2
  wires:
  Mux/1 -> Magnitude Squared/1, Switch/3, Normalization1/1
  v_e_x_in/1 -> Mux/1
  v_e_y_in/1 -> Mux/2
  Demux/1 -> v_e_x_out/1
  Demux/2 -> v_e_y_out/1
  Switch/1 -> Demux/1
  Product/1 -> Switch/1
  Magnitude Squared/1 -> Sum of Elements/1
  Sum of Elements/1 -> Sqrt/1
  max_v_hor_mps/1 -> Product/2, Subtract/1
  Sqrt/1 -> Subtract/2
  Normalization1/1 -> Product/1
  Subtract/1 -> Switch/2

== system torch_3dof_angle/WAYPOINT CONTROLLER/WP_NAV/heading_controller/heading_controller/heading_error ==
  heading_cmd_rad : Inport
  heading_rad : Inport  Port=2
  Abs : Abs  SaturateOnIntegerOverflow=off
  Compare To Constant : simulink/Logic and Bit Operations/Compare To Constant  relop=>  const=pi  OutDataTypeStr=boolean
  Constant : Constant  Value=2*pi  OutDataTypeStr=single
  Product : Product
  Sign : Signum
  Subtract : Sum  Inputs=+-
  Subtract1 : Sum  Inputs=+-
  Switch : Switch  Criteria=u2 > Threshold  SaturateOnIntegerOverflow=off  InputSameDT=off
  heading_error_rad : Outport
  wires:
  heading_cmd_rad/1 -> Subtract/1
  heading_rad/1 -> Subtract/2
  Subtract/1 -> Abs/1, Switch/3, Subtract1/1, Sign/1
  Compare To Constant/1 -> Switch/2
  Subtract1/1 -> Switch/1
  Switch/1 -> heading_error_rad/1
  Abs/1 -> Compare To Constant/1
  Sign/1 -> Product/1
  Product/1 -> Subtract1/2
  Constant/1 -> Product/2

== system torch_3dof_angle/determine arm and mode selection/Failsafe_management/Radio failsafe/Subsystem/Subsystem ==
  <incept_health_raw> : Inport
  Abs1 : Abs  SaturateOnIntegerOverflow=off
  Compare To Constant : simulink/Logic and Bit Operations/Compare To Constant  relop=>=  const=0.98  OutDataTypeStr=boolean
  e_stop counter : Subsystem
  incept_health_filter : Outport
  wires:
  Compare To Constant/1 -> e_stop counter/Enable
  Abs1/1 -> Compare To Constant/1
  <incept_health_raw>/1 -> e_stop counter/1(motor_e_stop_raw), Abs1/1
  e_stop counter/1(e_stop_filtered) -> incept_health_filter/1

== system torch_3dof_angle/POS_HOLD CONTROLLER/Horizontal speed controller/zero_vel_handling/Horizontal position controller/Horizontal_position_controller/convert to ve_cmd ==
  speed_cmd_mps : Inport
  bearing_to_target_rad : Inport  Port=2
  Cos : Trigonometry  Operator=cos
  Product : Product
  Product1 : Product
  Sin : Trigonometry
  ve_x_cmd : Outport
  ve_y_cmd : Outport  Port=2
  wires:
  Product/1 -> ve_x_cmd/1
  speed_cmd_mps/1 -> Product/1, Product1/1
  bearing_to_target_rad/1 -> Cos/1, Sin/1
  Cos/1 -> Product/2
  Sin/1 -> Product1/2
  Product1/1 -> ve_y_cmd/1

== system torch_3dof_angle/determine arm and mode selection/Failsafe_management/Radio failsafe/Subsystem/Subsystem/e_stop counter ==
  note: This is to ensure e_stop event is not triggered unless e_stop command is sent for more than 0.3 s to prevent false trigger
  motor_e_stop_raw : Inport
  Enable : EnablePort  StatesWhenEnabling=reset
  Compare To Constant : simulink/Logic and Bit Operations/Compare To Constant  relop=>=  const=0.5  OutDataTypeStr=boolean
  Discrete-Time Integrator : DiscreteIntegrator  SampleTime=framePeriod_s  LimitOutput=on  UpperSaturationLimit=1  LowerSaturationLimit=0  ICPrevOutput=DiscIntNeverNeededParam  ICPrevScaledInput=DiscIntNeverNeededParam
  Gain : Gain  Gain=2
  e_stop_filtered : Outport
  wires:
  Compare To Constant/1 -> e_stop_filtered/1
  Discrete-Time Integrator/1 -> Compare To Constant/1
  Gain/1 -> Discrete-Time Integrator/1
  motor_e_stop_raw/1 -> Gain/1

== matlab function torch_3dof_angle/command selection/mode_norm/remap ==
  data: raw_in input; norm_out output; in_min input; in_max input; out_min input; out_max input
function norm_out = remap(raw_in,in_min,in_max,out_min,out_max)
norm_out = (raw_in - in_min) * (out_max - out_min)/(in_max-in_min) + out_min;

== matlab function torch_3dof_angle/ANGLE CONTROLLER1/Pitch Controller/pitch_D_DLPF/MATLAB Function ==
  data: prev_val input; raw_val input; filtered_val output; freq_cut input; samp_freq input
function filtered_val = IIR_filt( prev_val,raw_val, freq_cut, samp_freq)
    fc = freq_cut/samp_freq;
    b = 2 - cos(2 * pi * fc) - sqrt((2 - cos(2 * pi * fc))^2 - 1);
    a = 1 - b;
    filtered_val = a * raw_val + b * prev_val;

== matlab function torch_3dof_angle/POS_HOLD CONTROLLER/Horizontal speed controller/Subsystem/roll_D_DLPF/MATLAB Function ==
  data: prev_val input; raw_val input; filtered_val output; freq_cut input; samp_freq input
function filtered_val = IIR_filt( prev_val,raw_val, freq_cut, samp_freq)
    fc = freq_cut/samp_freq;
    b = 2 - cos(2 * pi * fc) - sqrt((2 - cos(2 * pi * fc))^2 - 1);
    a = 1 - b;
    filtered_val = a * raw_val + b * prev_val;

== matlab function torch_3dof_angle/POS_HOLD CONTROLLER/Horizontal speed controller/Subsystem1/roll_D_DLPF/MATLAB Function ==
  data: prev_val input; raw_val input; filtered_val output; freq_cut input; samp_freq input
function filtered_val = IIR_filt( prev_val,raw_val, freq_cut, samp_freq)
    fc = freq_cut/samp_freq;
    b = 2 - cos(2 * pi * fc) - sqrt((2 - cos(2 * pi * fc))^2 - 1);
    a = 1 - b;
    filtered_val = a * raw_val + b * prev_val;

== matlab function torch_3dof_angle/Stab_input_conversion/remap from min_spin to max/remap1 ==
  data: raw_in input; norm_out output; in_min input; in_max input; out_min input; out_max input
function norm_out = remap(raw_in,in_min,in_max,out_min,out_max)
norm_out = (raw_in - in_min) * (out_max - out_min)/(in_max-in_min) + out_min;

== matlab function torch_3dof_angle/POS_HOLD CONTROLLER/Vertical speed controller/roll_D_DLPF/MATLAB Function ==
  data: prev_val input; raw_val input; filtered_val output; freq_cut input; samp_freq input
function filtered_val = IIR_filt( prev_val,raw_val, freq_cut, samp_freq)
    fc = freq_cut/samp_freq;
    b = 2 - cos(2 * pi * fc) - sqrt((2 - cos(2 * pi * fc))^2 - 1);
    a = 1 - b;
    filtered_val = a * raw_val + b * prev_val;

== matlab function torch_3dof_angle/cmd to raw pwm1/motor_PWM_denormalize/remap ==
  data: norm_in input; raw_out output; in_min input; in_max input; out_min input; out_max input
function raw_out = remap(norm_in,in_min,in_max,out_min,out_max)
raw_out = (norm_in - in_min) * (out_max - out_min)/(in_max-in_min) + out_min;

== matlab function torch_3dof_angle/ANGLE CONTROLLER1/Pitch Controller/pitch_input_DLPF/MATLAB Function ==
  data: prev_val input; raw_val input; filtered_val output; freq_cut input; samp_freq input
function filtered_val = IIR_filt( prev_val,raw_val, freq_cut, samp_freq)
    fc = freq_cut/samp_freq;
    b = 2 - cos(2 * pi * fc) - sqrt((2 - cos(2 * pi * fc))^2 - 1);
    a = 1 - b;
    filtered_val = a * raw_val + b * prev_val;

== matlab function torch_3dof_angle/POS_HOLD CONTROLLER/Vertical speed controller/Pitch_D_DLPF/MATLAB Function ==
  data: prev_val input; raw_val input; filtered_val output; freq_cut input
function filtered_val = IIR_filt( prev_val,raw_val, freq_cut)
    fc = freq_cut/100;
    b = 2 - cos(2 * pi * fc) - sqrt((2 - cos(2 * pi * fc))^2 - 1);
    a = 1 - b;
    filtered_val = a * raw_val + b * prev_val;

== matlab function torch_3dof_angle/WAYPOINT CONTROLLER/determine target/determine max speeds ==
  data: cur_tar_pos input; max_v_z_mps output; cur_pos input; max_hor_spd input; max_ver_spd input; max_v_xy_mps output
function [max_v_z_mps, max_v_xy_mps] = calc_speed_limits(cur_tar_pos, cur_pos, max_hor_spd, max_ver_spd)
    % Determine horz and vert speed limits to ensure that aircraft
    % arrives at WP at roughly the same time
    diff = cur_tar_pos - cur_pos;
    xy_mag = norm(diff(1:2)); % lateral dist
    time_to_vert = abs(diff(3) / max_ver_spd) + 1;
    %max_v_xy_mps = min([xy_mag / time_to_vert, max_hor_spd]);
    max_v_xy_mps = max_hor_spd;

    time_to_horz = (xy_mag / max_hor_spd) + 1;
    %max_v_z_mps = min([abs(diff(3)) / time_to_horz, max_ver_spd]);
    max_v_z_mps = max_ver_spd;

== matlab function torch_3dof_angle/WAYPOINT CONTROLLER CMD/pitch_norm_deadband/remap_with_deadband ==
  data: raw_in input; norm_out output; in_min input; in_max input; out_min input; out_max input; deadband input
function norm_out = remap_deadband(raw_in, in_min, in_max, out_min, out_max, deadband)
in_avg = (in_min + in_max) / 2;
out_avg = (out_min + out_max) / 2;

in_deadband_range = (in_max - in_min) * deadband / 2;
in_deadband_low = in_avg - in_deadband_range;
in_deadband_hi = in_avg + in_deadband_range;

if raw_in < in_deadband_low
    norm_out = (raw_in - in_deadband_low) .* (out_max - out_avg)./(in_deadband_low - in_min) + out_avg;
elseif raw_in > in_deadband_low && raw_in < in_deadband_hi
    norm_out = out_avg;
else
    norm_out = (raw_in - in_deadband_hi) .* (out_max - out_avg)./(in_max - in_deadband_hi) + out_avg;
end

== matlab function torch_3dof_angle/WAYPOINT CONTROLLER CMD/remap from min_spin to max/remap1 ==
  data: raw_in input; norm_out output; in_min input; in_max input; out_min input; out_max input
function norm_out = remap(raw_in,in_min,in_max,out_min,out_max)
norm_out = (raw_in - in_min) * (out_max - out_min)/(in_max-in_min) + out_min;

== matlab function torch_3dof_angle/WAYPOINT CONTROLLER/WP_NAV/Horizontal position controller/deviation_calc ==
  data: tar_pos input; cur_pos input; dev_dist_m output; prev_pos input; dev_bearing_rad output
function [dev_dist_m, dev_bearing_rad]  = fcn(tar_pos, cur_pos, prev_pos)
    % Input pos are the 2D NED position
    deviation_asix_bearing = atan2(tar_pos(2) - prev_pos(2), tar_pos(1) - prev_pos(1)) + pi/2;
    unit_deviation_vec = [cos(deviation_asix_bearing), sin(deviation_asix_bearing)];

    vec_tar_to_prev = tar_pos - prev_pos;
    vec_tar_to_cur = tar_pos - cur_pos;

    len_tar_to_cur = norm(vec_tar_to_cur(1:2));

    y = vec_tar_to_cur(2) * vec_tar_to_prev(1) - vec_tar_to_cur(1) * vec_tar_to_prev(2);
    x = vec_tar_to_prev(1) * vec_tar_to_cur(1) + vec_tar_to_prev(2) * vec_tar_to_cur(2);

    dev_vec = (y * len_tar_to_cur / sqrt(x^2 + y^2)) * unit_deviation_vec;
    dev_dist_m = norm(dev_vec);
    dev_bearing_rad = atan2(dev_vec(2), dev_vec(1));
end

== matlab function torch_3dof_angle/WAYPOINT CONTROLLER/determine target/determine_current_tar_pos ==
  data: fp_x input; cur_target_pos output; fp_y input; fp_z input; wp_frame input; home_lat_rad input; home_lon_rad input; home_alt input
function cur_target_pos = determine_current_tar_pos(fp_x, fp_y, fp_z, ...
                                                    wp_frame, home_lat_rad, home_lon_rad, home_alt)
% WP reference frames
% 1 - relative to armed position
% 2 - who knows
% 3 - abosulute. Using lat, lon, alt
% 4 - cage frame. WP are relative to cage origin
    if wp_frame == 3
        cur_target_pos = mission_item_to_ned(fp_x, fp_y, fp_z, home_lat_rad, home_lon_rad, home_alt);   
    elseif wp_frame == 4
        r2d = 180 / pi;
        cage_origin = [33.2154770, -87.5436600, 0];
        cage_home_pos_lla = [home_lat_rad * r2d, home_lon_rad * r2d, 0];
        cage_home_pos_ned = single(lla_to_ned(cage_home_pos_lla, cage_origin));
        cur_target_pos = single([fp_x; -fp_y; -fp_z]) - cage_home_pos_ned;
    else
        cur_target_pos = single([0; 0; 0]);
    end
end

== matlab function torch_3dof_angle/WAYPOINT CONTROLLER/wp_completion_check/check_wp_reached ==
  data: target_pos input; reached output boolean; ned_pos input; Aircraft_Control_wp_radius input
function reached = check_wp_reached(target_pos, ned_pos, Aircraft_Control_wp_radius)

diff = target_pos - ned_pos;
reached = norm(diff) <= Aircraft_Control_wp_radius;
